simulink model "InverterGyro"  (R2020a)
settings: Solver=ode23tb  StartTime=0.0  StopTime=10.0  MaxStep=Tc
values from neighbouring files (symbols this model uses):
  cp = 40    [LD9_29rpm38.m]
  CTRPIFF_CLIP_RELEASE = 0.05    [InverterGyro_Init.m]
  emf_fb_p = 0.2*k    (= 0.4)    [LD9_29rpm38.m]
  emf_p = 0.08*k    (= 0.16)    [LD9_29rpm38.m]
  emf_valid = 0.25e3    (= 250)    [LD9_29rpm38.m]
  fcut_u_stack_flt = 161    [InverterGyro_Init.m]
  g0 = fcut_u_stack_flt * Tcontrol_INV    (= 0.0268333333333)    [InverterGyro_Init.m]
  g1 = 1 - g0    (= 0.973166666667)    [InverterGyro_Init.m]
  Ibez = In*sqrt(2)    [LD9_29rpm38.m]
  iq_lim = 1.4    [InverterGyro_Init.m]
  J = J    [plant_data.m]
  kalman_gamma = 1.6    [LD9_29rpm38.m]
  kalman_iq_est = 0    [LD9_29rpm38.m]
  kalman_w = kalman_gamma/k    (= 0.32)    [LD9_29rpm38.m]
  ki_inv_d = 18    [InverterGyro_Init.m]
  ki_inv_q = 18    [InverterGyro_Init.m]
  ki_w = 35    [InverterGyro_Init.m]
  kp_inv_d = 2    [InverterGyro_Init.m]
  kp_inv_q = 2    [InverterGyro_Init.m]
  kp_w = 8    [InverterGyro_Init.m]
  La = 1/3*(Lq+Ld)    (= 0.00188)    [LD9_29rpm38.m]
  Lb = 1/3*(Lq-Ld)    (= 0.00028)    [LD9_29rpm38.m]
  Ld_norm = Ld/Lbez    [LD9_29rpm38.m]
  LFi_0 = LFi_d/10    (= 8e-06)    [InverterGyro_Init.m]
  LFi_d = 80e-6    (= 8e-05)    [InverterGyro_Init.m]
  Ll = 5e-6    (= 5e-06)    [LD9_29rpm38.m]
  Lq_norm = Lq/Lbez    [LD9_29rpm38.m]
  Ls_norm = Ls/Lbez    [LD9_29rpm38.m]
  motorc_m_scale = 2/3*Vdc_nom/Ubez    [LD9_29rpm38.m]
  Omega_bez_motor = we_motor    (= 123.066656217)    [LD9_29rpm38.m]
  Omega_bez_plant = Omega_bez_motor * plant_motor_ratio    (= 123.066656217)    [LD9_29rpm38.m]
  Omega_bez_plant_m = Omega_bez_motor_m * plant_motor_ratio    (= 3.07666640542)    [LD9_29rpm38.m]
  phi = Ubez/Omega_bez_plant    [LD9_29rpm38.m]
  RLFi_0 = RLFi_d/3    (= 0.000334933333333)    [InverterGyro_Init.m]
  RLFi_d = 157*0.08*LFi_d    (= 0.0010048)    [InverterGyro_Init.m]
  Rs = 3.15e-3*n_modules    (= 0.0126)    [LD9_29rpm38.m]
  Rs_norm = Rs/Xbez    [LD9_29rpm38.m]
  settle_time = 0.1    [InverterGyro_Init.m]
  sign_speed = 1    [InverterGyro_Init.m]
  spdobs_emf_o_fact = 0    [LD9_29rpm38.m]
  spdobs_emf_q_fact = 0    [LD9_29rpm38.m]
  Tc = 1e-5    (= 1e-05)    [InverterGyro_Init.m]
  Tcontrol_INV = 1/fPWM_INV/2    (= 0.000166666666667)    [InverterGyro_Init.m]
  Tintcom = 100e-3    (= 0.1)    [InverterGyro_Init.m]
  Tload = 0.75*Tnom    (= 60750)    [LD9_29rpm38.m]
  Tnom = 324e3/n_modules    (= 81000)    [LD9_29rpm38.m]
  tref = 2    [InverterGyro_Init.m]
  Tsamp = Tc    (= 1e-05)    [InverterGyro_Init.m]
  udc_min = 0.85    [InverterGyro_Init.m]
  Vdc_nom = Vdc_ref    (= 720)    [InverterGyro_Init.m]    (also in LD9_29rpm38.m = Vdc_ref)
  Vdc_ref = 720    [InverterGyro_Init.m]
  wref = Omega_sim    [InverterGyro_Init.m]
undefined symbols (not defined in the file or in its folder): magnitude
libraries: powerlib x31, simulink x4, simulink_extras x4, cstblocks x1
(part 2 of 2)

== system InverterGyro/PSM/PSM: Electrical System/dq2alphabeta/dq-alphabeta ==
  note: va=V cos(wt)
      | vb=V cos(wt-2pi/3)
      | vc=V cos(wt+2pi/3)
  d : Inport
  q : Inport  Port=2
  wt : Inport  Port=3
  Product{,1..3} (4 alike) : Product  RndMeth=Zero
  Sum : Sum  Inputs=+-
  Sum1 : Sum
  Trigonometric Function : Trigonometry  Operator=cos
  Trigonometric Function1 : Trigonometry
  alpha : Outport
  beta : Outport  Port=2
  wires:
  wt/1 -> Trigonometric Function1/1, Trigonometric Function/1
  Trigonometric Function/1 -> [cos]
  Trigonometric Function1/1 -> [sin]
  [cos] -> Product/1
  d/1 -> Product/2, Product2/2
  Product/1 -> Sum/1
  Product1/1 -> Sum/2
  [sin] -> Product1/1
  q/1 -> Product1/2, Product3/2
  Sum/1 -> alpha/1
  [sin] -> Product2/1
  Product2/1 -> Sum1/1
  Product3/1 -> Sum1/2
  [cos] -> Product3/1
  Sum1/1 -> beta/1

== system InverterGyro/PSM/PSM: Electrical System/invLmat/Luu ==
  wt : Inport
  Constant : Constant  Value=La
  Constant1 : Constant  Value=Lb
  Constant2 : Constant  Value=Ll
  Gain1 : Gain  Gain=2
  Product : Product
  Sum1 : Sum  Inputs=+++
  Trigonometric Function : Trigonometry  Operator=cos
  Luu : Outport
  wires:
  Gain1/1 -> Trigonometric Function/1
  Trigonometric Function/1 -> Product/2
  Sum1/1 -> Luu/1
  Constant1/1 -> Product/1
  wt/1 -> Gain1/1
  Product/1 -> Sum1/3
  Constant/1 -> Sum1/2
  Constant2/1 -> Sum1/1

== system InverterGyro/PSM/PSM: Electrical System/invLmat/Luv ==
  wt : Inport
  Constant : Constant  Value=La
  Constant1 : Constant  Value=Lb
  Constant2 : Constant  Value=-2*pi/3
  Gain1 : Gain  Gain=2
  Gain2 : Gain  Gain=-1/2
  Product : Product
  Sum1 : Sum  Inputs=|++
  Sum2 : Sum  Inputs=|++
  Trigonometric Function : Trigonometry  Operator=cos
  Luv : Outport
  wires:
  wt/1 -> Gain1/1
  Constant1/1 -> Product/1
  Sum1/1 -> Luv/1
  Trigonometric Function/1 -> Product/2
  Product/1 -> Sum1/2
  Constant/1 -> Gain2/1
  Gain2/1 -> Sum1/1
  Gain1/1 -> Sum2/1
  Sum2/1 -> Trigonometric Function/1
  Constant2/1 -> Sum2/2

== system InverterGyro/PSM/PSM: Electrical System/invLmat/Luw ==
  wt : Inport
  Constant : Constant  Value=La
  Constant1 : Constant  Value=Lb
  Constant2 : Constant  Value=2*pi/3
  Gain1 : Gain  Gain=2
  Gain2 : Gain  Gain=-1/2
  Product : Product
  Sum1 : Sum  Inputs=|++
  Sum2 : Sum  Inputs=|++
  Trigonometric Function : Trigonometry  Operator=cos
  Luw : Outport
  wires:
  Constant2/1 -> Sum2/2
  Sum2/1 -> Trigonometric Function/1
  Gain1/1 -> Sum2/1
  Gain2/1 -> Sum1/1
  Constant/1 -> Gain2/1
  Product/1 -> Sum1/2
  Trigonometric Function/1 -> Product/2
  Sum1/1 -> Luw/1
  Constant1/1 -> Product/1
  wt/1 -> Gain1/1

== system InverterGyro/PSM/PSM: Electrical System/invLmat/Lvv ==
  wt : Inport
  Constant : Constant  Value=La
  Constant1 : Constant  Value=Lb
  Constant2 : Constant  Value=2*pi/3
  Constant3 : Constant  Value=Ll
  Gain1 : Gain  Gain=2
  Product : Product
  Sum1 : Sum  Inputs=+++
  Sum2 : Sum  Inputs=|++
  Trigonometric Function : Trigonometry  Operator=cos
  Lvv : Outport
  wires:
  wt/1 -> Gain1/1
  Constant1/1 -> Product/1
  Sum1/1 -> Lvv/1
  Trigonometric Function/1 -> Product/2
  Product/1 -> Sum1/3
  Constant/1 -> Sum1/2
  Gain1/1 -> Sum2/1
  Sum2/1 -> Trigonometric Function/1
  Constant2/1 -> Sum2/2
  Constant3/1 -> Sum1/1

== system InverterGyro/PSM/PSM: Electrical System/invLmat/Lvw ==
  wt : Inport
  Constant : Constant  Value=La
  Constant1 : Constant  Value=Lb
  Constant2 : Constant  Value=2*pi
  Gain1 : Gain  Gain=2
  Gain2 : Gain  Gain=-1/2
  Product : Product
  Sum1 : Sum  Inputs=|++
  Sum2 : Sum  Inputs=|++
  Trigonometric Function : Trigonometry  Operator=cos
  Lvw : Outport
  wires:
  wt/1 -> Gain1/1
  Constant1/1 -> Product/1
  Sum1/1 -> Lvw/1
  Trigonometric Function/1 -> Product/2
  Product/1 -> Sum1/2
  Constant/1 -> Gain2/1
  Gain2/1 -> Sum1/1
  Gain1/1 -> Sum2/1
  Sum2/1 -> Trigonometric Function/1
  Constant2/1 -> Sum2/2

== system InverterGyro/PSM/PSM: Electrical System/invLmat/Lww ==
  wt : Inport
  Constant : Constant  Value=La
  Constant1 : Constant  Value=Lb
  Constant2 : Constant  Value=-2*pi/3
  Constant3 : Constant  Value=Ll
  Gain1 : Gain  Gain=2
  Product : Product
  Sum1 : Sum  Inputs=+++
  Sum2 : Sum  Inputs=|++
  Trigonometric Function : Trigonometry  Operator=cos
  Lww : Outport
  wires:
  Constant2/1 -> Sum2/2
  Sum2/1 -> Trigonometric Function/1
  Gain1/1 -> Sum2/1
  Constant/1 -> Sum1/2
  Product/1 -> Sum1/3
  Trigonometric Function/1 -> Product/2
  Sum1/1 -> Lww/1
  Constant1/1 -> Product/1
  wt/1 -> Gain1/1
  Constant3/1 -> Sum1/1

== system InverterGyro/INVERTER/INVERTER Control/PSM Control/Current control/PI D ==
  id_tilde : Inport
  clip : Inport  Port=2
  1/Ti : Gain  Gain=kp_inv_d  SaturateOnIntegerOverflow=on  OutDataTypeStr=Inherit: Same as input  ParamDataTypeStr=Inherit: Same as input
  Constant : Constant  Value=0
  Sum2 : Sum  Inputs=+-  SaturateOnIntegerOverflow=on
  Sum4 : Sum  SaturateOnIntegerOverflow=on
  Sum5 : Sum  SaturateOnIntegerOverflow=on
  Sum8 : Sum  SaturateOnIntegerOverflow=on
  Switch1 : Switch  Threshold=0.5
  Switch2 : Switch  Threshold=0.5
  To Workspace2 : ToWorkspace  VariableName=Vds_ff  SampleTime=Tsamp
      settings: MaxDataPoints=Nc
  To Workspace3 : ToWorkspace  VariableName=Vds_ctrl  SampleTime=Tsamp
      settings: MaxDataPoints=Nc
  To Workspace5 : ToWorkspace  VariableName=Vds_ctrl_out  SampleTime=Tsamp
      settings: MaxDataPoints=Nc
  Unit Delay1 : UnitDelay  SampleTime=Tcontrol_INV  HasFrameUpgradeWarning=on
  Unit Delay2 : UnitDelay  SampleTime=Tcontrol_INV  HasFrameUpgradeWarning=on
  kp1 : Gain  Gain=CTRPIFF_CLIP_RELEASE*Tcontrol_INV  SaturateOnIntegerOverflow=on  OutDataTypeStr=Inherit: Same as input  ParamDataTypeStr=Inherit: Same as input
  kp2 : Gain  Gain=ki_inv_d*Tcontrol_INV  SaturateOnIntegerOverflow=on  OutDataTypeStr=Inherit: Same as input  ParamDataTypeStr=Inherit: Same as input
  Vds_out : Outport
  wires:
  [vd_ff] -> Sum8/2, To Workspace2/1
  id_tilde/1 -> kp2/1, 1/Ti/1
  Sum8/1 -> To Workspace5/1, Vds_out/1  "vd_out"
  Switch1/1 -> Unit Delay2/1
  Sum4/1 -> Sum5/2, Switch1/3
  kp1/1 -> Sum2/2
  Sum2/1 -> Switch1/1
  Unit Delay2/1 -> Sum4/2, kp1/1, Sum2/1
  1/Ti/1 -> Sum5/1
  Sum5/1 -> To Workspace3/1, Sum8/1
  Switch2/1 -> Sum4/1
  kp2/1 -> Switch2/3
  clip/1 -> Unit Delay1/1
  [clip] -> Switch2/2
  [clip] -> Switch1/2
  Constant/1 -> Switch2/1
  Unit Delay1/1 -> [clip]

== system InverterGyro/INVERTER/INVERTER Control/PSM Control/Current control/PI Q ==
  iq_tilde : Inport
  clip : Inport  Port=2
  1/Ti : Gain  Gain=kp_inv_q  SaturateOnIntegerOverflow=on  OutDataTypeStr=Inherit: Same as input  ParamDataTypeStr=Inherit: Same as input
  Constant : Constant  Value=0
  Sum2 : Sum  Inputs=+-  SaturateOnIntegerOverflow=on
  Sum4 : Sum  SaturateOnIntegerOverflow=on
  Sum5 : Sum  SaturateOnIntegerOverflow=on
  Sum8 : Sum  SaturateOnIntegerOverflow=on
  Switch1 : Switch  Threshold=0.5
  Switch2 : Switch  Threshold=0.5
  To Workspace2 : ToWorkspace  VariableName=Vqs_ff  SampleTime=Tsamp
      settings: MaxDataPoints=Nc
  To Workspace3 : ToWorkspace  VariableName=Vqs_ctrl  SampleTime=Tsamp
      settings: MaxDataPoints=Nc
  To Workspace5 : ToWorkspace  VariableName=Vqs_ctrl_out  SampleTime=Tsamp
      settings: MaxDataPoints=Nc
  Unit Delay1 : UnitDelay  SampleTime=Tcontrol_INV  HasFrameUpgradeWarning=on
  Unit Delay2 : UnitDelay  SampleTime=Tcontrol_INV  HasFrameUpgradeWarning=on
  kp1 : Gain  Gain=CTRPIFF_CLIP_RELEASE*Tcontrol_INV  SaturateOnIntegerOverflow=on  OutDataTypeStr=Inherit: Same as input  ParamDataTypeStr=Inherit: Same as input
  kp2 : Gain  Gain=ki_inv_q*Tcontrol_INV  SaturateOnIntegerOverflow=on  OutDataTypeStr=Inherit: Same as input  ParamDataTypeStr=Inherit: Same as input
  Vqs_out : Outport
  wires:
  Constant/1 -> Switch2/1
  [clip] -> Switch1/2
  [clip] -> Switch2/2
  clip/1 -> Unit Delay1/1
  kp2/1 -> Switch2/3
  Switch2/1 -> Sum4/1
  Sum5/1 -> Sum8/1, To Workspace3/1
  1/Ti/1 -> Sum5/1
  Unit Delay2/1 -> Sum2/1, kp1/1, Sum4/2
  Sum2/1 -> Switch1/1
  kp1/1 -> Sum2/2
  Sum4/1 -> Sum5/2, Switch1/3
  Switch1/1 -> Unit Delay2/1
  Sum8/1 -> To Workspace5/1, Vqs_out/1  "vq_out"
  iq_tilde/1 -> 1/Ti/1, kp2/1
  [vq_ff] -> Sum8/2, To Workspace2/1
  Unit Delay1/1 -> [clip]

== system InverterGyro/INVERTER/INVERTER Control/PSM Control/Current control/bounder1 ==
  vd : Inport
  k_sat : Inport  Port=2
  length : Inport  Port=3
  Constant : Constant
  Constant1 : Constant  Value=0
  Divide : Product
  Switch : Switch  Threshold=sqrt(3)/2
  Switch1 : Switch  Threshold=sqrt(3)/2
  To Workspace1 : ToWorkspace  VariableName=Vds_not_clipped  SampleTime=Tsamp
      settings: MaxDataPoints=Nc
  To Workspace7 : ToWorkspace  VariableName=Vds_clipped  SampleTime=Tsamp
      settings: MaxDataPoints=Nc
  vd_sat : Outport
  clip : Outport  Port=2
  wires:
  vd/1 -> To Workspace1/1, Switch1/3, Divide/2
  k_sat/1 -> Divide/1
  Divide/1 -> To Workspace7/1, Switch1/1
  Switch1/1 -> vd_sat/1
  Switch/1 -> clip/1
  length/1 -> Switch/2, Switch1/2
  Constant/1 -> Switch/1
  Constant1/1 -> Switch/3

== system InverterGyro/INVERTER/INVERTER Control/PSM Control/Current control/bounder2 ==
  length : Inport
  k_sat : Inport  Port=2
  vq : Inport  Port=3
  Constant : Constant
  Constant1 : Constant  Value=0
  Divide : Product
  Switch : Switch  Threshold=sqrt(3)/2
  Switch1 : Switch  Threshold=sqrt(3)/2
  To Workspace1 : ToWorkspace  VariableName=Vqs_not_clipped  SampleTime=Tsamp
      settings: MaxDataPoints=Nc
  To Workspace7 : ToWorkspace  VariableName=Vqs_clipped  SampleTime=Tsamp
      settings: MaxDataPoints=Nc
  vq_sat : Outport
  clip : Outport  Port=2
  wires:
  Constant1/1 -> Switch/3
  Constant/1 -> Switch/1
  length/1 -> Switch1/2, Switch/2
  Switch/1 -> clip/1
  Switch1/1 -> vq_sat/1
  Divide/1 -> Switch1/1, To Workspace7/1
  k_sat/1 -> Divide/1
  vq/1 -> Divide/2, Switch1/3, To Workspace1/1

== system InverterGyro/INVERTER/INVERTER Control/PSM Control/Current control/feedback linearization ==
  id : Inport
  iq : Inport  Port=2
  wm : Inport  Port=3
  Divide1 : Product
  Divide2 : Product
  Gain1 : Gain  Gain=Lq_norm
  Gain2 : Gain
  Gain3 : Gain  Gain=Ld_norm
  Gain4 : Gain
  Sum12 : Sum  SaturateOnIntegerOverflow=on
  Sum6 : Sum  Inputs=-+  SaturateOnIntegerOverflow=on
  Out1 : Outport
  Out2 : Outport  Port=2
  wires:
  Divide1/1 -> Gain3/1
  iq/1 -> Divide2/1  "iq"
  wm/1 -> Divide2/2, Divide1/1  "omega"
  Divide2/1 -> Gain1/1
  id/1 -> Divide1/2  "id"
  [emf_d] -> Sum6/2
  [emf_q] -> Sum12/1
  Sum6/1 -> Gain4/1
  Sum12/1 -> Gain2/1
  Gain2/1 -> Out2/1  "vq_ff"
  Gain4/1 -> Out1/1  "vd_ff"
  Gain1/1 -> Sum6/1
  Gain3/1 -> Sum12/2

== system InverterGyro/INVERTER/INVERTER Control/PSM Control/Current control/switch ==
  clip 1 : Inport
  clip 2 : Inport  Port=2
  Constant4 : Constant
  Constant5 : Constant  Value=0
  Sum1 : Sum  SaturateOnIntegerOverflow=on
  Switch : Switch  Threshold=0.5
  clip : Outport
  wires:
  Constant5/1 -> Switch/3
  Switch/1 -> clip/1
  Constant4/1 -> Switch/1
  Sum1/1 -> Switch/2
  clip 1/1 -> Sum1/1
  clip 2/1 -> Sum1/2

== system InverterGyro/INVERTER/INVERTER Control/PSM Control/Current control/vector lenght ==
  md : Inport
  mq : Inport  Port=2
  1/Ti3 : Gain  Gain=sqrt(3)/2  SaturateOnIntegerOverflow=on  OutDataTypeStr=Inherit: Same as input  ParamDataTypeStr=Inherit: Same as input
  Math Function : Math  Operator=magnitude^2  SignedPower=on  SaturateOnIntegerOverflow=on
  Math Function1 : Math  Operator=magnitude^2  SignedPower=on  SaturateOnIntegerOverflow=on
  Math Function2 : Math  Operator=reciprocal  SignedPower=on  SaturateOnIntegerOverflow=on
  Sqrt : Sqrt  SaturateOnIntegerOverflow=on
  Sum5 : Sum  SaturateOnIntegerOverflow=on
  k_sat : Outport
  m : Outport  Port=2
  wires:
  Math Function2/1 -> 1/Ti3/1
  Sqrt/1 -> m/1, Math Function2/1  "length"
  mq/1 -> Math Function1/1  "q"
  Math Function1/1 -> Sum5/2
  Math Function/1 -> Sum5/1
  Sum5/1 -> Sqrt/1
  1/Ti3/1 -> k_sat/1  "k_sat"
  md/1 -> Math Function/1  "d"

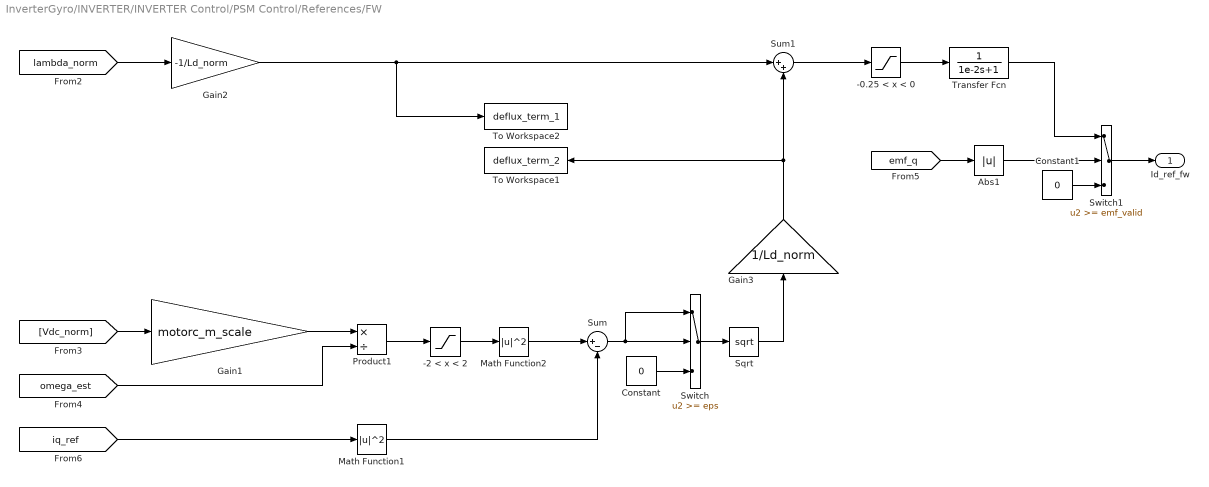
== system InverterGyro/INVERTER/INVERTER Control/PSM Control/References/FW ==
  -0.25 < x < 0 : Saturate  UpperLimit=0  LowerLimit=-0.25  LinearizeAsGain=off
  -2 < x < 2 : Saturate  UpperLimit=2  LowerLimit=-2
  Abs1 : Abs
  Constant : Constant  Value=0
  Constant1 : Constant  Value=0
  Gain1 : Gain  Gain=motorc_m_scale
  Gain2 : Gain  Gain=-1/Ld_norm
  Gain3 : Gain  Gain=1/Ld_norm
  Math Function1 : Math  Operator=magnitude^2  SignedPower=on  SaturateOnIntegerOverflow=on
  Math Function2 : Math  Operator=magnitude^2  SignedPower=on  SaturateOnIntegerOverflow=on
  Product1 : Product  Inputs=*/  RndMeth=Zero
  Sqrt : Sqrt  SaturateOnIntegerOverflow=on
  Sum : Sum  Inputs=|+-
  Sum1 : Sum  Inputs=|++
  Switch : Switch  Threshold=eps
  Switch1 : Switch  Threshold=emf_valid
  To Workspace1 : ToWorkspace  VariableName=deflux_term_2  SampleTime=Tsamp
      settings: MaxDataPoints=Nc
  To Workspace2 : ToWorkspace  VariableName=deflux_term_1  SampleTime=Tsamp
      settings: MaxDataPoints=Nc
  Transfer Fcn : TransferFcn  Denominator=[1e-2 1]
  Id_ref_fw : Outport
  wires:
  -0.25 < x < 0/1 -> Transfer Fcn/1
  Sqrt/1 -> Gain3/1
  Math Function1/1 -> Sum/2
  Sum1/1 -> -0.25 < x < 0/1
  Gain2/1 -> To Workspace2/1, Sum1/1
  Math Function2/1 -> Sum/1
  Gain1/1 -> Product1/1
  Product1/1 -> -2 < x < 2/1
  -2 < x < 2/1 -> Math Function2/1
  Sum/1 -> Switch/1, Switch/2
  Switch/1 -> Sqrt/1
  Constant/1 -> Switch/3
  Gain3/1 -> To Workspace1/1, Sum1/2
  [emf_q] -> Abs1/1
  Abs1/1 -> Switch1/2
  Constant1/1 -> Switch1/3
  Switch1/1 -> Id_ref_fw/1
  Transfer Fcn/1 -> Switch1/1
  [lambda_norm] -> Gain2/1
  [Vdc_norm] -> Gain1/1
  [iq_ref] -> Math Function1/1
  [omega_est] -> Product1/2

== system InverterGyro/INVERTER/INVERTER Control/PSM Control/References/MTPA ==
  -1 < x < 0 : Saturate  UpperLimit=0  LowerLimit=-1
  0 < x < 2 : Saturate  UpperLimit=2  LowerLimit=0
  Abs : Abs
  Divide : Product  Inputs=*/
  Gain1 : Gain  Gain=(1/(Lq_norm - Ld_norm)/2)^2
  Gain2 : Gain  Gain=1/(Lq_norm - Ld_norm)/2
  Math Function : Math  Operator=magnitude^2  SignedPower=on  SaturateOnIntegerOverflow=on
  Math Function1 : Math  Operator=magnitude^2  SignedPower=on  SaturateOnIntegerOverflow=on
  Sqrt : Sqrt  SaturateOnIntegerOverflow=on
  Sum : Sum  Inputs=|++
  Sum1 : Sum  Inputs=|+-
  To Workspace4 : ToWorkspace  VariableName=lambda_norm_calc  SampleTime=Tsamp
      settings: MaxDataPoints=Nc
  u_stack_flt : Subsystem
  Id_ref_mtpa : Outport
  tag scope: lambda_norm=global
  wires:
  Gain1/1 -> Sum/1
  [lambda_norm] -> Gain2/1
  Sum1/1 -> -1 < x < 0/1
  Math Function1/1 -> Sum/2
  Gain2/1 -> Sum1/1
  [lambda_norm] -> Math Function/1
  Math Function/1 -> Gain1/1
  Sqrt/1 -> Sum1/2
  -1 < x < 0/1 -> Id_ref_mtpa/1
  Sum/1 -> Sqrt/1
  [iq_ref] -> Math Function1/1
  Abs/1 -> 0 < x < 2/1
  [omega_est] -> Divide/2
  0 < x < 2/1 -> To Workspace4/1, [lambda_norm]
  [emf_q] -> Divide/1
  Divide/1 -> Abs/1

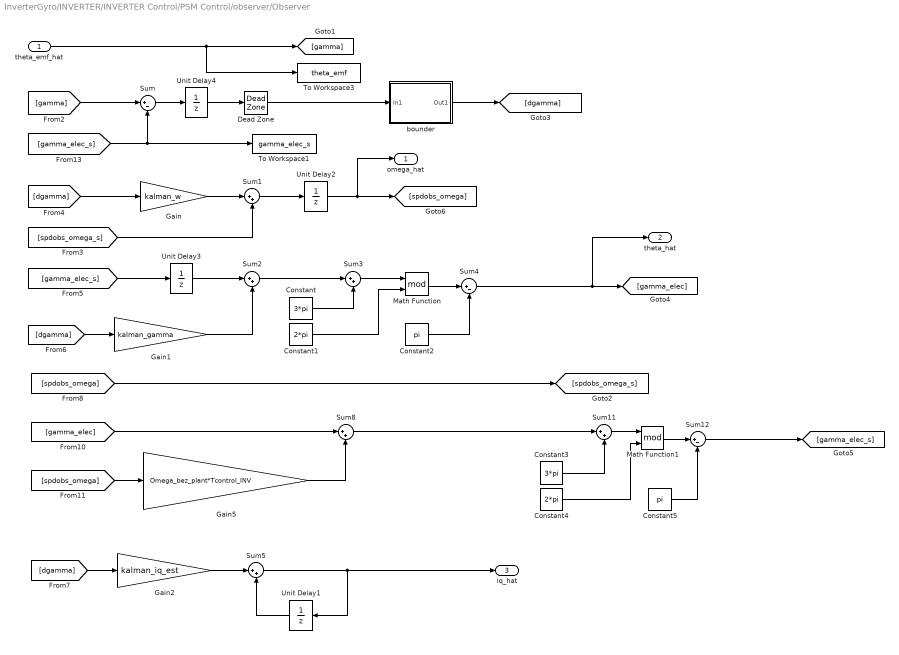
== system InverterGyro/INVERTER/INVERTER Control/PSM Control/observer/Observer ==
  theta_emf_hat : Inport
  Constant : Constant  Value=3*pi
  Constant1 : Constant  Value=2*pi
  Constant2 : Constant  Value=pi
  Constant3 : Constant  Value=3*pi
  Constant4 : Constant  Value=2*pi
  Constant5 : Constant  Value=pi
  Dead Zone : DeadZone  LowerValue=-0.000001  UpperValue=0.000001  SaturateOnIntegerOverflow=on
  Gain : Gain  Gain=kalman_w
  Gain1 : Gain  Gain=kalman_gamma
  Gain2 : Gain  Gain=kalman_iq_est
  Gain5 : Gain  Gain=Omega_bez_plant*Tcontrol_INV
  Math Function : Math  Operator=mod  SignedPower=on  SaturateOnIntegerOverflow=on
  Math Function1 : Math  Operator=mod  SignedPower=on  SaturateOnIntegerOverflow=on
  Sum : Sum  Inputs=|+-
  Sum{1..3,5,8,11} (6 alike) : Sum  Inputs=|++
  Sum12 : Sum  Inputs=|+-
  Sum4 : Sum  Inputs=|+-
  To Workspace1 : ToWorkspace  VariableName=gamma_elec_s  SampleTime=Tsamp
      settings: MaxDataPoints=Nc
  To Workspace3 : ToWorkspace  VariableName=theta_emf  SampleTime=Tsamp
      settings: MaxDataPoints=Nc
  Unit Delay1 : UnitDelay  SampleTime=Tcontrol_INV  HasFrameUpgradeWarning=on
  Unit Delay2 : UnitDelay  InitialCondition=eps  SampleTime=Tcontrol_INV  HasFrameUpgradeWarning=on
  Unit Delay3 : UnitDelay  InitialCondition=eps  SampleTime=Tcontrol_INV  HasFrameUpgradeWarning=on
  Unit Delay4 : UnitDelay  SampleTime=Tcontrol_INV  HasFrameUpgradeWarning=on
  bounder : Subsystem
  omega_hat : Outport
  theta_hat : Outport  Port=2
  iq_hat : Outport  Port=3
  wires:
  theta_emf_hat/1 -> To Workspace3/1, [gamma]
  Sum/1 -> Unit Delay4/1
  [dgamma] -> Gain/1
  [spdobs_omega_s] -> Sum1/2
  Gain/1 -> Sum1/1
  [dgamma] -> Gain1/1
  Sum2/1 -> Sum3/1
  Constant/1 -> Sum3/2
  Constant1/1 -> Math Function/2
  Sum3/1 -> Math Function/1
  Math Function/1 -> Sum4/1
  Constant2/1 -> Sum4/2
  [gamma_elec_s] -> Unit Delay3/1
  [dgamma] -> Gain2/1
  Gain2/1 -> Sum5/1
  Unit Delay1/1 -> Sum5/2
  [spdobs_omega] -> [spdobs_omega_s]
  [gamma_elec] -> Sum8/1
  [spdobs_omega] -> Gain5/1
  Gain5/1 -> Sum8/2
  Constant3/1 -> Sum11/2
  Constant4/1 -> Math Function1/2
  Sum11/1 -> Math Function1/1
  Math Function1/1 -> Sum12/1
  Constant5/1 -> Sum12/2
  Sum8/1 -> Sum11/1
  Gain1/1 -> Sum2/2
  Sum12/1 -> [gamma_elec_s]
  Sum4/1 -> [gamma_elec], theta_hat/1
  Sum1/1 -> Unit Delay2/1
  Unit Delay2/1 -> [spdobs_omega], omega_hat/1
  [gamma] -> Sum/1
  [gamma_elec_s] -> To Workspace1/1, Sum/2
  Unit Delay4/1 -> Dead Zone/1
  Unit Delay3/1 -> Sum2/1
  Dead Zone/1 -> bounder/1(In1)
  bounder/1(Out1) -> [dgamma]
  Sum5/1 -> iq_hat/1, Unit Delay1/1

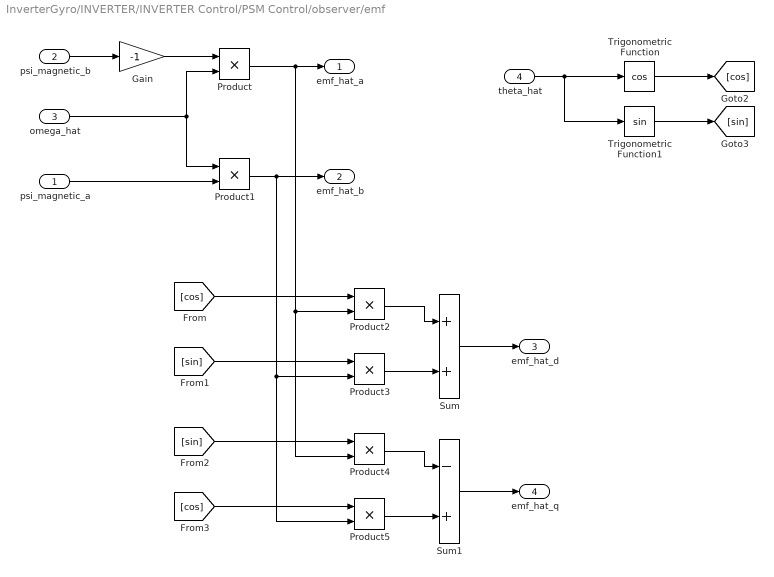
== system InverterGyro/INVERTER/INVERTER Control/PSM Control/observer/emf ==
  psi_magnetic_a : Inport
  psi_magnetic_b : Inport  Port=2
  omega_hat : Inport  Port=3
  theta_hat : Inport  Port=4
  Gain : Gain  Gain=-1
  Product{,1..5} (6 alike) : Product  RndMeth=Zero
  Sum : Sum
  Sum1 : Sum  Inputs=-+
  Trigonometric Function : Trigonometry  Operator=cos
  Trigonometric Function1 : Trigonometry
  emf_hat_a : Outport
  emf_hat_b : Outport  Port=2
  emf_hat_d : Outport  Port=3
  emf_hat_q : Outport  Port=4
  wires:
  psi_magnetic_b/1 -> Gain/1
  Gain/1 -> Product/1
  Product/1 -> Product4/2, Product2/2, emf_hat_a/1
  omega_hat/1 -> Product/2, Product1/1
  Product1/1 -> Product5/2, Product3/2, emf_hat_b/1
  psi_magnetic_a/1 -> Product1/2
  theta_hat/1 -> Trigonometric Function1/1, Trigonometric Function/1
  Trigonometric Function/1 -> [cos]
  Trigonometric Function1/1 -> [sin]
  Sum1/1 -> emf_hat_q/1
  [cos] -> Product5/1
  Product5/1 -> Sum1/2
  Product4/1 -> Sum1/1
  [sin] -> Product4/1
  Sum/1 -> emf_hat_d/1
  [sin] -> Product3/1
  Product3/1 -> Sum/2
  Product2/1 -> Sum/1
  [cos] -> Product2/1

== system InverterGyro/INVERTER/INVERTER Control/PSM Control/observer/psi_stator_alpha_hat ==
  v_s : Inport
  i_s : Inport  Port=2
  Gain1 : Gain  Gain=Rs_norm
  Gain2 : Gain  Gain=emf_fb_p
  Gain3 : Gain  Gain=emf_p
  Gain4 : Gain  Gain=Omega_bez_plant*Tcontrol_INV
  Gain5 : Gain  Gain=Ls_norm
  Gain6 : Gain  Gain=motorc_m_scale
  Product : Product  RndMeth=Zero
  Sum : Sum  Inputs=|+-
  Sum1 : Sum  Inputs=|+-
  Sum2 : Sum  Inputs=++-  SaturateOnIntegerOverflow=on
  Sum3 : Sum  Inputs=|++
  Sum4 : Sum  Inputs=+-  SaturateOnIntegerOverflow=on
  Unit Delay1 : UnitDelay  SampleTime=Tcontrol_INV  HasFrameUpgradeWarning=on
  Unit Delay2 : UnitDelay  SampleTime=Tcontrol_INV  HasFrameUpgradeWarning=on
  psi_stator : Outport
  psi_magnetic : Outport  Port=2
  wires:
  [psi_m_a] -> Sum1/1
  [psi_magnetic_a] -> Sum1/2
  Gain4/1 -> Sum3/1
  Sum2/1 -> Gain4/1
  Gain3/1 -> Sum2/3
  i_s/1 -> Gain5/1, Gain1/1  "i"
  Gain1/1 -> Sum/2
  Sum/1 -> Sum2/2
  v_s/1 -> Product/1  "v"
  Gain5/1 -> Sum4/2
  Sum4/1 -> Unit Delay2/1
  Unit Delay1/1 -> Gain3/1, Sum3/2
  Sum3/1 -> Sum4/1, Unit Delay1/1, psi_stator/1
  Unit Delay2/1 -> psi_magnetic/1
  Sum1/1 -> Gain2/1
  Gain2/1 -> Sum2/1
  Gain6/1 -> Sum/1
  [Vdc_norm] -> Product/2
  Product/1 -> Gain6/1

== system InverterGyro/INVERTER/INVERTER Control/PSM Control/observer/psi_stator_beta_hat ==
  v_s : Inport
  i_s : Inport  Port=2
  Gain1 : Gain  Gain=Rs_norm
  Gain2 : Gain  Gain=emf_fb_p
  Gain3 : Gain  Gain=emf_p
  Gain4 : Gain  Gain=Omega_bez_plant*Tcontrol_INV
  Gain5 : Gain  Gain=Ls_norm
  Gain6 : Gain  Gain=motorc_m_scale
  Product : Product  RndMeth=Zero
  Sum : Sum  Inputs=|+-
  Sum1 : Sum  Inputs=|+-
  Sum2 : Sum  Inputs=++-  SaturateOnIntegerOverflow=on
  Sum3 : Sum  Inputs=|++
  Sum4 : Sum  Inputs=+-  SaturateOnIntegerOverflow=on
  Unit Delay1 : UnitDelay  SampleTime=Tcontrol_INV  HasFrameUpgradeWarning=on
  Unit Delay2 : UnitDelay  SampleTime=Tcontrol_INV  HasFrameUpgradeWarning=on
  psi_stator : Outport
  psi_magnetic : Outport  Port=2
  wires:
  Sum4/1 -> Unit Delay2/1
  Gain5/1 -> Sum4/2
  Sum/1 -> Sum2/2
  Gain1/1 -> Sum/2
  i_s/1 -> Gain1/1, Gain5/1  "i"
  Gain3/1 -> Sum2/3
  Sum2/1 -> Gain4/1
  Gain4/1 -> Sum3/1
  Sum1/1 -> Gain2/1
  [psi_magnetic_b] -> Sum1/2
  [psi_m_b] -> Sum1/1
  Unit Delay1/1 -> Sum3/2, Gain3/1
  Sum3/1 -> Sum4/1, Unit Delay1/1, psi_stator/1
  Unit Delay2/1 -> psi_magnetic/1
  Gain2/1 -> Sum2/1
  v_s/1 -> Product/1  "v"
  [Vdc_norm] -> Product/2
  Product/1 -> Gain6/1
  Gain6/1 -> Sum/1

== system InverterGyro/INVERTER/INVERTER Control/PSM Control/observer/theta_emf_hat_calc ==
  phi_magnetic_a : Inport
  psi_magnetic_b : Inport  Port=2
  Abs : Abs
  Gain : Gain  Gain=spdobs_emf_q_fact
  Gain1 : Gain  Gain=spdobs_emf_o_fact
  Gain2 : Gain  Gain=1/fcut_u_stack_flt
  Gain3 : Gain  Gain=1/2/pi
  Gain4 : Gain  Gain=Omega_bez_motor
  LTI System : cstblocks/LTI System  sys=fof1_z  IC=[]
  Selector : Selector  InputPortWidth=2  IndexOptions=Index vector (dialog)  Indices=[2]  OutputSizes=1
  Sum : Sum  Inputs=|++
  Sum1 : Sum  Inputs=|++
  Sum2 : Sum  Inputs=++|
  Switch : Switch  Threshold=emf_valid
  Trigonometric Function : Trigonometry  Operator=atan2
  Trigonometric Function1 : Trigonometry  Operator=atan
  theta_hat : Outport
  wires:
  psi_magnetic_b/1 -> Trigonometric Function/1
  phi_magnetic_a/1 -> Trigonometric Function/2
  [omega_est] -> Switch/1
  Switch/1 -> Gain1/1
  [omega_encoder] -> Switch/3
  Abs/1 -> Switch/2
  [idq] -> Selector/1
  Selector/1 -> LTI System/1
  LTI System/1 -> Gain/1
  Sum/1 -> Sum1/1
  Sum1/1 -> theta_hat/1
  Gain/1 -> Sum/2
  Gain1/1 -> Sum1/2
  Trigonometric Function/1 -> Sum2/2
  Sum2/1 -> Sum/1
  Gain2/1 -> Trigonometric Function1/1
  Gain3/1 -> Gain2/1
  Gain4/1 -> Gain3/1
  [omega_est] -> Gain4/1
  [emf_q] -> Abs/1

== system InverterGyro/INVERTER/INVERTER Control/PSM Control/References/MTPA/u_stack_flt ==
  input : Inport
  Gain3 : Gain  Gain=g1
  Gain6 : Gain  Gain=g0
  Sum : Sum  Inputs=|++
  Unit Delay1 : UnitDelay  SampleTime=Tcontrol_INV  HasFrameUpgradeWarning=on
  output : Outport
  wires:
  Sum/1 -> output/1, Unit Delay1/1
  Gain3/1 -> Sum/2
  Unit Delay1/1 -> Gain3/1
  input/1 -> Gain6/1
  Gain6/1 -> Sum/1

== system InverterGyro/INVERTER/INVERTER Control/PSM Control/observer/Observer/bounder ==
  In1 : Inport
  Compare To Constant : simulink/Logic and Bit Operations/Compare To Constant  relop=>  const=pi  OutDataTypeStr=boolean
  Compare To Constant1 : simulink/Logic and Bit Operations/Compare To Constant  relop=<  const=-pi  OutDataTypeStr=boolean
  Enabled Subsystem : Subsystem  TreatAsAtomicUnit=on
  Enabled Subsystem1 : Subsystem  TreatAsAtomicUnit=on
  Enabled Subsystem2 : Subsystem  TreatAsAtomicUnit=on
  Logical Operator : Logic  Operator=NOR  AllPortsSameDT=off  OutDataTypeStr=boolean
  Sum1 : Sum  Inputs=+++
  Out1 : Outport
  wires:
  In1/1 -> Enabled Subsystem2/1(In1), Enabled Subsystem1/1(In1), Enabled Subsystem/1(In1), Compare To Constant1/1, Compare To Constant/1
  Compare To Constant/1 -> Enabled Subsystem/Enable, Logical Operator/1
  Compare To Constant1/1 -> Enabled Subsystem1/Enable, Logical Operator/2
  Logical Operator/1 -> Enabled Subsystem2/Enable
  Enabled Subsystem/1(Out1) -> Sum1/1
  Enabled Subsystem2/1(Out1) -> Sum1/2
  Enabled Subsystem1/1(Out1) -> Sum1/3
  Sum1/1 -> Out1/1

== system InverterGyro/INVERTER/INVERTER Control/PSM Control/observer/Observer/bounder/Enabled Subsystem ==
  In1 : Inport
  Enable : EnablePort
  Constant : Constant  Value=2*pi
  Sum1 : Sum  Inputs=|+-
  Out1 : Outport
  wires:
  In1/1 -> Sum1/1
  Sum1/1 -> Out1/1
  Constant/1 -> Sum1/2

== system InverterGyro/INVERTER/INVERTER Control/PSM Control/observer/Observer/bounder/Enabled Subsystem1 ==
  In1 : Inport
  Enable : EnablePort
  Constant : Constant  Value=2*pi
  Sum1 : Sum  Inputs=|++
  Out1 : Outport
  wires:
  Constant/1 -> Sum1/2
  In1/1 -> Sum1/1
  Sum1/1 -> Out1/1

== system InverterGyro/INVERTER/INVERTER Control/PSM Control/observer/Observer/bounder/Enabled Subsystem2 ==
  In1 : Inport
  Enable : EnablePort
  Out1 : Outport
  wires:
  In1/1 -> Out1/1
